simulink model "ofdm_pktdetector_mimo"  (Simulink 6.6)
settings: Solver=ode45  StartTime=0.0  StopTime=simTime  RelTol=1e-3
PreLoadFcn:
  | init
PostLoadFcn:
  | init
InitFcn:
  | init
StartFcn:
  | init
undefined symbols (not defined in the file or in its folder): gcbh, xlBlockLoadCallback, xlGetSimulinkPeriod
libraries: xbsIndex_r4 x201
(part 1 of 3)
settings Model: Creator=murphpo  LastModifiedBy=CMC
settings DebuggingCC: SignalResolutionControl=TryResolveAllWithWarning  MultiTaskDSMMsg=warning  MultiTaskCondExecSysMsg=none
settings RTWCC: IncludeERTFirstTime=on

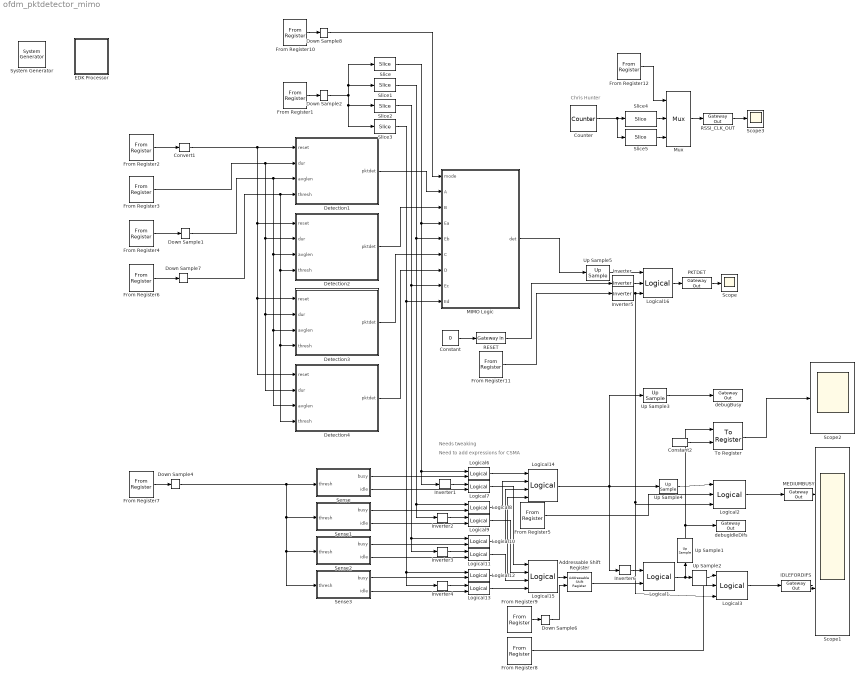
== system ofdm_pktdetector_mimo ==
  note: Chris Hunter
  note: Need to add expressions for CSMA
  note: Needs tweaking
  " System Generator" : xbsIndex_r4/ System Generator  Tag=genX  SystemSampleTime=-1  xilinxfamily=virtex2p  part=xc2vp70  speed=-6  package=ff1517  synthesis_tool=XST  clock_wrapper=Clock Enables  directory=./plb46_pktDet_v01  testbench=off  simulink_period=1/4  sysclk_period=10  dcm_input_clock_period=100  incr_netlist=off  trim_vbits=Everywhere in SubSystem  dbl_ovrd=According to Block Masks  core_generation=According to Block Masks  run_coregen=off  deprecated_control=off  eval_field=0  block_type=sysgen
      settings: block_version=8.2
  Addressable Shift Register : xbsIndex_r4/Addressable Shift Register  infer_latency=on  depth=2  initVector=[0]  en=off  dbl_ovrd=off  use_behavioral_HDL=off  use_rpm=off  block_type=addrsr
      settings: block_version=8.2
      settings: infoedit=|
      | Delay of  configurable length.  Any element  in the delay
      |     line   can    be   addressed   and   driven    onto   the   output
      |     port.<P><P>Hardware  notes: Implemented  using SRL16s.
      |     If Virtex-4, Virtex-II or Spartan-3 devices are used, multiple SRLC16s are cascaded together.
  Constant : Constant  Value=0
  Constant2 : xbsIndex_r4/Constant  arith_type=Boolean  const=1  n_bits=1  bin_pt=0  explicit_period=off  period=1  equ=P=C  opselect=C  inp2=PCIN>>17  opr=+  inp1=P  carry=CIN  dbl_ovrd=off  block_type=constant
      settings: block_version=8.2
  Convert1 : xbsIndex_r4/Convert  arith_type=Boolean  n_bits=16  bin_pt=14  quantization=Truncate  overflow=Wrap  latency=0  dbl_ovrd=off  pipeline=off  block_type=convert
      settings: block_version=VER_STRING_GOES_HERE
  Counter : xbsIndex_r4/Counter  cnt_type=Free Running  cnt_to=Inf  operation=Up  start_count=0  cnt_by_val=1  arith_type=Unsigned  n_bits=2  bin_pt=0  load_pin=off  rst=off  en=off  explicit_period=on  period=2/4  dbl_ovrd=off  use_behavioral_HDL=off  use_rpm=off  block_type=counter
      settings: block_version=VER_STRING_GOES_HERE
  Detection1 : Subsystem
  Detection2 : Subsystem
  Detection3 : Subsystem
  Detection4 : Subsystem
  Down Sample{1..2,4,6..8} (6 alike) : xbsIndex_r4/Down Sample  sample_ratio=4  sample_phase="Last Value of Frame  (most efficient)"  en=off  latency=1  dbl_ovrd=off  block_type=dsamp
      settings: block_version=VER_STRING_GOES_HERE
  EDK Processor : Subsystem  LoadFcn=xlBlockLoadCallback(gcbh);  mask(Xilinx EDK Processor Block){mode=EDK pcore generation, xmp=, MemVisToProc=<qt bgcolor="#FFFFFF"><div><img src="C:\Xilinx_101\DSP_Tools\common\bin\..\..\sysgen\data\images\registerplus.gif"> &lt;&lt;csma_avgThresh&gt;&gt;<br></div><div><img src="C:\Xilinx_101\DSP_Tools\common\bin\..\..\sysgen\data\images\registerplus.gif"> &lt;&lt;csma_difsPeriod&gt;&gt;<br></div><div><img src="C:\Xilinx_101\DSP_Tools\common\bin\..\..\sysgen\data\images\registerplus.gif"> &lt;&lt;csma_enableBusy&gt;&gt;<br></div><div><img src="C:\Xilinx_101\DSP_Tools\common\bin\..\..\sysgen\data\images\registerplus.gif"> &lt;&lt;csma_enableIdle&gt;&gt;<br></div><div><img src="C:\Xilinx_101\DSP_Tools\common\bin\..\..\sysgen\data\images\registerplus.gif"> &lt;&lt;pktDet_avgLen&gt;&gt;<br></div><div><img src="C:\Xilinx_101\DSP_Tools\common\bin\..\..\sysgen\data\images\registerplus.gif"> &lt;&lt;pktDet_avgThresh&gt;&gt;<br></div><div><img src="C:\Xilinx_101\DSP_Tools\common\bin\..\..\sysgen\data\images\registerplus.gif"> &lt;&lt;pktDet_clkRatioSel&gt;&gt;<br></div><div><img src="C:\Xilinx_101\DSP_Tools\common\bin\..\..\sysgen\data\images\registerplus.gif"> &lt;&lt;pktDet_detectionMask&gt;&gt;<br></div><div><img src="C:\Xilinx_101\DSP_Tools\common\bin\..\..\sysgen\data\images\registerplus.gif"> &lt;&lt;pktDet_detectionMode&gt;&gt;<br></div><div><img src="C:\Xilinx_101\DSP_Tools\common\bin\..\..\sysgen\data\images\registerplus.gif"> &lt;&lt;pktDet_idleDifs&gt;&gt;<br></div><div><img src="C:\Xilinx_101\DSP_Tools\common\bin\..\..\sysgen\data\images\registerplus.gif"> &lt;&lt;pktDet_masterReset&gt;&gt;<br></div><div><img src="C:\Xilinx_101\DSP_Tools\common\bin\..\..\sysgen\data\images\registerplus.gif"> &lt;&lt;pktDet_reset&gt;&gt;<br></div><div><img src="C:\Xilinx_101\DSP_Tools\common\bin\..\..\sysgen\data\images\registerplus.gif"> &lt;&lt;pktDet_resetDuration&gt;&gt;<br></div></qt>, AvailableMemories=<empty>, portInterfaceTable={'exposed'=>[],'portdir'=>[],'portname'=>[],'shortname'=>[]}, bus_type_sgadvanced=, bus_type=PLB, baseaddr=0x80000000, baseaddr_lock_sgadvanced=, baseaddr_lock=off, dual_clock_sgadvanced=, dual_clock=off, ucf_file=, inheritDeviceType_sgadvanced=, inheritDeviceType=off, clock_name=plb, internalPortList={}, resetPolarity=0, memxtable={'mlist'=>['ofdm_pktdetector_mimo/From Register7','ofdm_pktdetector_mimo/From Register9','ofdm_pktdetector_mimo/From Register5','ofdm_pktdetector_mimo/From Register8','ofdm_pktdetector_mimo/From Register4','ofdm_pktdetector_mimo/From Register6','ofdm_pktdetector_mimo/From Register12','ofdm_pktdetector_mimo/From Register1','ofdm_pktdetector_mimo/From Register10','ofdm_pktdetector_mimo/To Register','ofdm_pktdetector_mimo/From Register2','ofdm_pktdetector_mimo/From Register11','ofdm_pktdetector_mimo/From Register3'],'mlname'=>['\'csma_avgThresh\'','\'csma_difsPeriod\'','\'csma_enableBusy\'','\'csma_enableIdle\'','\'pktDet_avgLen\'','\'pktDet_avgThresh\'','\'pktDet_clkRatioSel\'','\'pktDet_detectionMask\'','\'pktDet_detectionMode\'','\'pktDet_idleDifs\'','\'pktDet_masterReset\'','\'pktDet_reset\'','\'pktDet_resetDuration\''],'mlstate'=>[0.00000000000000000,0.00000000000000000,0.00000000000000000,0.00000000000000000,0.00000000000000000,0.00000000000000000,0.00000000000000000,0.00000000000000000,0.00000000000000000,0.00000000000000000,0.00000000000000000,0.00000000000000000,0.00000000000000000]}, procinfo={'xmliface'=>'Xilinx//microblaze//iface.xml'}, fslifaceports=[0,0], memmapdirty=off, blockname=, xpsintstyle=default, proc=, has_advanced_control=0, sggui_pos=20,20,383,441, block_type=edkprocessor, block_version=2.4, sg_icon_stat=62,64,-1,-1,white,blue,0,07734,right, sg_mask_display=|, sg_list_contents={'table'=>{'AvailableMemories'=>'popup(<empty>)','userSelections'=>{'AvailableMemories'=>'<empty>'}}}, sg_blockgui_xml=}
      mask sg_mask_display=|
      | fprintf('','COMMENT: begin icon graphics');
      | patch([0 62 62 0 ],[0 0 64 64 ],[0.77 0.82 0.91]);
      | patch([14 4 19 4 14 30 34 38 56 42 29 19 33 19 29 42 56 38 34 30 14 ],[8 18 33 48 58 58 54 58 58 44 57 47 33 19 9 22 8 8 12 8 8 ],[0.98 0.96 0.92]);
      | plot([0 62 62 0 0 ],[0 0 64 64 0 ]);
      | fprintf('','COMMENT: end icon graphics');
      | fprintf('','COMMENT: begin icon text');
      | fprintf('','COMMENT: end icon text');
      mask prompts: mode "Configure Processor for"; xmp "EDK Project"; MemVisToProc ""; AvailableMemories "Available Memories"; portInterfaceTable ""; bus_type_sgadvanced ""; bus_type "Bus Type"; baseaddr "Base Address"; baseaddr_lock_sgadvanced ""; baseaddr_lock "Lock"; dual_clock_sgadvanced ""; dual_clock "Dual Clocks"; ucf_file "Constraint file"; inheritDeviceType_sgadvanced ""; inheritDeviceType "Inherit Device Type"; clock_name ""; internalPortList ""; resetPolarity ""; memxtable ""; procinfo ""; fslifaceports ""; memmapdirty ""; blockname ""; xpsintstyle ""; proc ""; has_advanced_control ""; sggui_pos ""; block_type ""; block_version ""; sg_icon_stat ""; sg_mask_display ""; sg_list_contents ""; sg_blockgui_xml ""
      mask help: Xilinx EDK Processor
      mask init:
      | try
      |   tmp_gcb = gcb;
      |   tmp_gcbh = gcbh;
      |   if (strcmp('SysGenIndex',get_param(bdroot(tmp_gcbh),'tag')) && ~isempty(regexp(bdroot(tmp_gcb), '^xbs', 'once')))
      |     return;
      |   end;
      |   xlMungeMaskParams;
      |   serialized_declarations = '{}';
      |   xledkprocessor_init();
      |   ptable_ = xlblockprep(get_param(tmp_gcb, 'MaskWSVariables'));
      | catch
      |   global dbgsysgen;
      |   if(~isempty(dbgsysgen) && dbgsysgen)
      |     e = regexprep(lasterr, '\n', '\nError: ');
      |     disp(['Error: While running MaskInit code on block ' tmp_gcb ': ' e]);
      |     error(e);
      |   end
      | end
      settings: CopyFcn=xlProcBlockCopyCallback(gcbh);xlBlockMoveCallback(gcbh);  DeleteFcn=xlDestroyGui(gcbh);  ModelCloseFcn=xlDestroyGui(gcbh);  PreSaveFcn=xlBlockPreSaveCallback(gcbh);  PostSaveFcn=xlBlockPostSaveCallback(gcbh);  DestroyFcn=xlDestroyGui(gcbh);  OpenFcn=bh=gcbh;xlProcBlockCallbacks('populatesharedmemorylistbox',bh);xlOpenGui(bh, 'edkprocessor_gui.xml', @xlProcBlockEnablement, @xlProcBlockAction)  CloseFcn=xlDestroyGui(gcbh);  MoveFcn=xlBlockMoveCallback(gcbh);
      mask Help: eval('');xlDoc('-book','sysgen','-topic','EDK_Processor');
      mask StyleString: popup(EDK pcore generation|HDL netlisting),edit,edit,popup(<empty>),edit,edit,popup(PLB|FSL),edit,edit,checkbox,edit,checkbox,edit,edit,checkbox,edit,edit,edit,edit,edit,edit,edit,edit,edit,edit,edit,edit,edit,edit,edit,edit,edit,edit
      mask Display:
      | fprintf('','COMMENT: begin icon graphics');
      | patch([0 62 62 0 ],[0 0 64 64 ],[0.77 0.82 0.91]);
      | patch([14 4 19 4 14 30 34 38 56 42 29 19 33 19 29 42 56 38 34 30 14 ],[8 18 33 48 58 58 54 58 58 44 57 47 33 19 9 22 8 8 12 8 8 ],[0.98 0.96 0.92]);
      | plot([0 62 62 0 0 ],[0 0 64 64 0 ]);
      | fprintf('','COMMENT: end icon graphics');
      | fprintf('','COMMENT: begin icon text');
      | disp('MicroBlaze');
      | 
      | fprintf('','COMMENT: end icon text');
  From Register1 : xbsIndex_r4/From Register  shared_memory_name='pktDet_detectionMask'  init=3  period=1/4  ownership=Locally owned and initialized  arith_type=Unsigned  n_bits=4  bin_pt=0  dbl_ovrd=off  block_type=fromreg
      settings: AttributesFormatString=From Register\n<< %<shared_memory_name> >>  infoedit="Register block that reads data to a shared memory register.  Delay of one sample period."  block_version=8.2
  From Register10 : xbsIndex_r4/From Register  shared_memory_name='pktDet_detectionMode'  init=1  period=1/4  ownership=Locally owned and initialized  arith_type=Unsigned  n_bits=1  bin_pt=0  dbl_ovrd=off  block_type=fromreg
      settings: AttributesFormatString=From Register\n<< %<shared_memory_name> >>  infoedit="Register block that reads data to a shared memory register.  Delay of one sample period."  block_version=8.2
  From Register11 : xbsIndex_r4/From Register  shared_memory_name='pktDet_reset'  init=0  period=1/4  ownership=Locally owned and initialized  arith_type=Unsigned  n_bits=1  bin_pt=0  dbl_ovrd=off  block_type=fromreg
      settings: AttributesFormatString=From Register\n<< %<shared_memory_name> >>  infoedit="Register block that reads data to a shared memory register.  Delay of one sample period."  block_version=8.2
  From Register12 : xbsIndex_r4/From Register  shared_memory_name='pktDet_clkRatioSel'  init=0  period=1/4  ownership=Locally owned and initialized  arith_type=Unsigned  n_bits=1  bin_pt=0  dbl_ovrd=off  block_type=fromreg
      settings: AttributesFormatString=From Register\n<< %<shared_memory_name> >>  infoedit="Register block that reads data to a shared memory register.  Delay of one sample period."  block_version=8.2
  From Register2 : xbsIndex_r4/From Register  shared_memory_name='pktDet_masterReset'  init=0  period=1/4  ownership=Locally owned and initialized  arith_type=Unsigned  n_bits=1  bin_pt=0  dbl_ovrd=off  block_type=fromreg
      settings: AttributesFormatString=From Register\n<< %<shared_memory_name> >>  infoedit="Register block that reads data to a shared memory register.  Delay of one sample period."  block_version=8.2
  From Register3 : xbsIndex_r4/From Register  shared_memory_name='pktDet_resetDuration'  init=resetDuration  period=1/4  ownership=Locally owned and initialized  arith_type=Unsigned  n_bits=16  bin_pt=0  dbl_ovrd=off  block_type=fromreg
      settings: AttributesFormatString=From Register\n<< %<shared_memory_name> >>  infoedit="Register block that reads data to a shared memory register.  Delay of one sample period."  block_version=8.2
  From Register4 : xbsIndex_r4/From Register  shared_memory_name='pktDet_avgLen'  init=2^5  period=1/4  ownership=Locally owned and initialized  arith_type=Unsigned  n_bits=5  bin_pt=0  dbl_ovrd=off  block_type=fromreg
      settings: AttributesFormatString=From Register\n<< %<shared_memory_name> >>  infoedit="Register block that reads data to a shared memory register.  Delay of one sample period."  block_version=8.2
  From Register5 : xbsIndex_r4/From Register  shared_memory_name='csma_enableBusy'  init=1  period=1/4  ownership=Locally owned and initialized  arith_type=Unsigned  n_bits=1  bin_pt=0  dbl_ovrd=off  block_type=fromreg
      settings: AttributesFormatString=From Register\n<< %<shared_memory_name> >>  infoedit="Register block that reads data to a shared memory register.  Delay of one sample period."  block_version=8.2
  From Register6 : xbsIndex_r4/From Register  shared_memory_name='pktDet_avgThresh'  init=avgMode_avgThresh  period=1/4  ownership=Locally owned and initialized  arith_type=Unsigned  n_bits=16  bin_pt=0  dbl_ovrd=off  block_type=fromreg
      settings: AttributesFormatString=From Register\n<< %<shared_memory_name> >>  infoedit="Register block that reads data to a shared memory register.  Delay of one sample period."  block_version=8.2
  From Register7 : xbsIndex_r4/From Register  shared_memory_name='csma_avgThresh'  init=avgMode_avgThresh  period=1/4  ownership=Locally owned and initialized  arith_type=Unsigned  n_bits=16  bin_pt=0  dbl_ovrd=off  block_type=fromreg
      settings: AttributesFormatString=From Register\n<< %<shared_memory_name> >>  infoedit="Register block that reads data to a shared memory register.  Delay of one sample period."  block_version=8.2
  From Register8 : xbsIndex_r4/From Register  shared_memory_name='csma_enableIdle'  init=1  period=1/4  ownership=Locally owned and initialized  arith_type=Unsigned  n_bits=1  bin_pt=0  dbl_ovrd=off  block_type=fromreg
      settings: AttributesFormatString=From Register\n<< %<shared_memory_name> >>  infoedit="Register block that reads data to a shared memory register.  Delay of one sample period."  block_version=8.2
  From Register9 : xbsIndex_r4/From Register  shared_memory_name='csma_difsPeriod'  init=625  period=1/4  ownership=Locally owned and initialized  arith_type=Unsigned  n_bits=10  bin_pt=0  dbl_ovrd=off  block_type=fromreg
      settings: AttributesFormatString=From Register\n<< %<shared_memory_name> >>  infoedit="Register block that reads data to a shared memory register.  Delay of one sample period."  block_version=8.2
  IDLEFORDIFS : xbsIndex_r4/Gateway Out  hdl_port=on  timing_constraint=None  locs_specified=off  LOCs={}  block_type=gatewayout
      settings: infoedit="Gateway out block.  Converts Xilinx fixed point inputs into ouputs of type Simulink integer, double, or fixed point.<P><P>Hardware notes:  In hardware these blocks become top level output ports or are discarded, depending on how they are configured."  block_version=VER_STRING_GOES_HERE
  Inverter{,1..6} (7 alike) : xbsIndex_r4/Inverter  en=off  latency=0  dbl_ovrd=off  block_type=inv
      settings: block_version=8.2
  Logical{1,6,8,10,12} (5 alike) : xbsIndex_r4/Logical  logical_function=AND  inputs=2  en=off  latency=0  precision=Full  arith_type=Unsigned  n_bits=16  bin_pt=0  align_bp=on  dbl_ovrd=off  block_type=logical
      settings: block_version=8.2
  Logical{7,9,11,13} (4 alike) : xbsIndex_r4/Logical  logical_function=OR  inputs=2  en=off  latency=0  precision=Full  arith_type=Unsigned  n_bits=16  bin_pt=0  align_bp=on  dbl_ovrd=off  block_type=logical
      settings: block_version=8.2
  Logical14 : xbsIndex_r4/Logical  logical_function=OR  inputs=4  en=off  latency=0  precision=Full  arith_type=Unsigned  n_bits=16  bin_pt=0  align_bp=on  dbl_ovrd=off  block_type=logical
      settings: block_version=8.2
  Logical15 : xbsIndex_r4/Logical  logical_function=AND  inputs=4  en=off  latency=0  precision=Full  arith_type=Unsigned  n_bits=16  bin_pt=0  align_bp=on  dbl_ovrd=off  block_type=logical
      settings: block_version=8.2
  Logical16 : xbsIndex_r4/Logical  logical_function=AND  inputs=3  en=off  latency=0  precision=Full  arith_type=Unsigned  n_bits=16  bin_pt=0  align_bp=on  dbl_ovrd=off  block_type=logical
      settings: block_version=8.2
  Logical2 : xbsIndex_r4/Logical  logical_function=AND  inputs=3  en=off  latency=0  precision=Full  arith_type=Unsigned  n_bits=16  bin_pt=0  align_bp=on  dbl_ovrd=off  block_type=logical
      settings: block_version=8.2
  Logical3 : xbsIndex_r4/Logical  logical_function=AND  inputs=3  en=off  latency=0  precision=Full  arith_type=Unsigned  n_bits=16  bin_pt=0  align_bp=on  dbl_ovrd=off  block_type=logical
      settings: block_version=8.2
  MEDIUMBUSY : xbsIndex_r4/Gateway Out  hdl_port=on  timing_constraint=None  locs_specified=off  LOCs={}  block_type=gatewayout
      settings: infoedit="Gateway out block.  Converts Xilinx fixed point inputs into ouputs of type Simulink integer, double, or fixed point.<P><P>Hardware notes:  In hardware these blocks become top level output ports or are discarded, depending on how they are configured."  block_version=VER_STRING_GOES_HERE
  MIMO Logic : Subsystem
  Mux : xbsIndex_r4/Mux  inputs=2  en=off  latency=0  precision=Full  arith_type=Unsigned  n_bits=16  bin_pt=14  quantization=Truncate  overflow=Wrap  dbl_ovrd=off  block_type=mux
      settings: block_version=8.2.02
  PKTDET : xbsIndex_r4/Gateway Out  hdl_port=on  timing_constraint=None  locs_specified=off  LOCs={}  block_type=gatewayout
      settings: infoedit="Gateway out block.  Converts Xilinx fixed point inputs into ouputs of type Simulink integer, double, or fixed point.<P><P>Hardware notes:  In hardware these blocks become top level output ports or are discarded, depending on how they are configured."  block_version=VER_STRING_GOES_HERE
  RESET : xbsIndex_r4/Gateway In  arith_type=Unsigned  n_bits=1  bin_pt=0  quantization="Round  (unbiased: +/- Inf)"  overflow=Saturate  period=1/4  dbl_ovrd=off  timing_constraint=None  locs_specified=off  LOCs={}  block_type=gatewayin
      settings: infoedit="Gateway in block.  Converts inputs of type Simulink integer, double and fixed point to  Xilinx fixed point type.<P><P>Hardware notes:  In hardware these blocks become top level input ports."  block_version=VER_STRING_GOES_HERE
  RSSI_CLK_OUT : xbsIndex_r4/Gateway Out  hdl_port=on  timing_constraint=None  locs_specified=off  LOCs={}  block_type=gatewayout
      settings: infoedit="Gateway out block.  Converts Xilinx fixed point inputs into ouputs of type Simulink integer, double, or fixed point.<P><P>Hardware notes:  In hardware these blocks become top level output ports or are discarded, depending on how they are configured."  block_version=VER_STRING_GOES_HERE
  Scope : Scope
  Scope1 : Scope  NumInputPorts=2
      settings: YMin=-5~-5  YMax=5~5  SaveName=ScopeData2
  Scope2 : Scope
      settings: SaveName=ScopeData4
  Scope3 : Scope
      settings: SaveName=ScopeData3
  Sense : Subsystem
  Sense1 : Subsystem
  Sense2 : Subsystem
  Sense3 : Subsystem
  Slice : xbsIndex_r4/Slice  nbits=1  boolean_output=off  mode=Lower Bit Location + Width  bit1=0  base1=MSB of Input  bit0=0  base0=LSB of Input  dbl_ovrd=off  block_type=slice
      settings: infoedit="Extracts a given range of bits from each input sample and presents it at the output.  The output type is ordinarily unsigned with binary point at zero, but can be Boolean when the slice is one bit wide.<P><P>Hardware notes: In hardware this block costs nothing."  block_version=8.2
  Slice1 : xbsIndex_r4/Slice  nbits=1  boolean_output=off  mode=Lower Bit Location + Width  bit1=0  base1=MSB of Input  bit0=1  base0=LSB of Input  dbl_ovrd=off  block_type=slice
      settings: infoedit="Extracts a given range of bits from each input sample and presents it at the output.  The output type is ordinarily unsigned with binary point at zero, but can be Boolean when the slice is one bit wide.<P><P>Hardware notes: In hardware this block costs nothing."  block_version=8.2
  Slice2 : xbsIndex_r4/Slice  nbits=1  boolean_output=off  mode=Lower Bit Location + Width  bit1=0  base1=MSB of Input  bit0=2  base0=LSB of Input  dbl_ovrd=off  block_type=slice
      settings: infoedit="Extracts a given range of bits from each input sample and presents it at the output.  The output type is ordinarily unsigned with binary point at zero, but can be Boolean when the slice is one bit wide.<P><P>Hardware notes: In hardware this block costs nothing."  block_version=8.2
  Slice3 : xbsIndex_r4/Slice  nbits=1  boolean_output=off  mode=Lower Bit Location + Width  bit1=0  base1=MSB of Input  bit0=3  base0=LSB of Input  dbl_ovrd=off  block_type=slice
      settings: infoedit="Extracts a given range of bits from each input sample and presents it at the output.  The output type is ordinarily unsigned with binary point at zero, but can be Boolean when the slice is one bit wide.<P><P>Hardware notes: In hardware this block costs nothing."  block_version=8.2
  Slice4 : xbsIndex_r4/Slice  nbits=1  boolean_output=off  mode=Lower Bit Location + Width  bit1=0  base1=MSB of Input  bit0=0  base0=LSB of Input  dbl_ovrd=off  block_type=slice
      settings: infoedit="Extracts a given range of bits from each input sample and presents it at the output.  The output type is ordinarily unsigned with binary point at zero, but can be Boolean when the slice is one bit wide.<P><P>Hardware notes: In hardware this block costs nothing."  block_version=8.2.02
  Slice5 : xbsIndex_r4/Slice  nbits=1  boolean_output=off  mode=Upper Bit Location + Width  bit1=0  base1=MSB of Input  bit0=0  base0=LSB of Input  dbl_ovrd=off  block_type=slice
      settings: infoedit="Extracts a given range of bits from each input sample and presents it at the output.  The output type is ordinarily unsigned with binary point at zero, but can be Boolean when the slice is one bit wide.<P><P>Hardware notes: In hardware this block costs nothing."  block_version=8.2.02
  To Register : xbsIndex_r4/To Register  shared_memory_name='pktDet_idleDifs'  init=0  ownership=Locally owned and initialized  explicit_data_type=on  arith_type=Unsigned  n_bits=1  bin_pt=0  dbl_ovrd=off  block_type=toreg
      settings: AttributesFormatString=To Register\n<< %<shared_memory_name> >>  infoedit="Register block that writes data to a shared memory register.  Delay of one sample period."  block_version=8.2
  Up Sample1 : xbsIndex_r4/Up Sample  Orientation=up  sample_ratio=4  copy_samples=on  dbl_ovrd=off  block_type=usamp
      settings: infoedit="Up samples input data.  Inserted values  can be zeros or copies of the most recent input sample.<P><P>Hardware notes: No hardware is needed if inserted values are copies of the input sample; otherwise, a mux and single bit flip-flop are used."  block_version=8.2
  Up Sample{2..5} (4 alike) : xbsIndex_r4/Up Sample  sample_ratio=4  copy_samples=on  dbl_ovrd=off  block_type=usamp
      settings: infoedit="Up samples input data.  Inserted values  can be zeros or copies of the most recent input sample.<P><P>Hardware notes: No hardware is needed if inserted values are copies of the input sample; otherwise, a mux and single bit flip-flop are used."  block_version=8.2
  debugBusy : xbsIndex_r4/Gateway Out  hdl_port=on  timing_constraint=None  locs_specified=off  LOCs={}  block_type=gatewayout
      settings: infoedit="Gateway out block.  Converts Xilinx fixed point inputs into ouputs of type Simulink integer, double, or fixed point.<P><P>Hardware notes:  In hardware these blocks become top level output ports or are discarded, depending on how they are configured."  block_version=VER_STRING_GOES_HERE
  debugIdleDifs : xbsIndex_r4/Gateway Out  hdl_port=on  timing_constraint=None  locs_specified=off  LOCs={}  block_type=gatewayout
      settings: infoedit="Gateway out block.  Converts Xilinx fixed point inputs into ouputs of type Simulink integer, double, or fixed point.<P><P>Hardware notes:  In hardware these blocks become top level output ports or are discarded, depending on how they are configured."  block_version=VER_STRING_GOES_HERE
  wires:
  From Register4/1 -> Down Sample1/1
  RSSI_CLK_OUT/1 -> Scope3/1
  From Register2/1 -> Convert1/1
  From Register6/1 -> Down Sample7/1
  Convert1/1 -> Detection1/1(reset), Detection3/1(reset), Detection4/1(reset), Detection2/1(reset)
  From Register3/1 -> Detection1/2(dur), Detection3/2(dur), Detection4/2(dur), Detection2/2(dur)
  Down Sample1/1 -> Detection1/3(avglen), Detection3/3(avglen), Detection4/3(avglen), Detection2/3(avglen)
  Down Sample7/1 -> Detection1/4(thresh), Detection3/4(thresh), Detection4/4(thresh), Detection2/4(thresh)
  From Register1/1 -> Down Sample2/1
  Down Sample2/1 -> Slice/1, Slice1/1, Slice2/1, Slice3/1
  MIMO Logic/1(det) -> Up Sample5/1
  Slice/1 -> Logical6/1, Inverter1/1, MIMO Logic/4(Ea)
  Slice1/1 -> Logical8/1, Inverter2/1, MIMO Logic/5(Eb)
  Slice2/1 -> Logical10/1, Inverter3/1, MIMO Logic/8(Ec)
  Slice3/1 -> Logical12/1, Inverter4/1, MIMO Logic/9(Ed)
  PKTDET/1 -> Scope/1
  RESET/1 -> Inverter/1
  Constant/1 -> RESET/1
  Up Sample5/1 -> Logical16/1
  Logical16/1 -> PKTDET/1
  From Register7/1 -> Down Sample4/1
  Down Sample4/1 -> Sense/1(thresh), Sense2/1(thresh), Sense3/1(thresh), Sense1/1(thresh)
  Sense/1(busy) -> Logical6/2
  Sense/2(idle) -> Logical7/2
  Sense1/1(busy) -> Logical8/2
  Sense1/2(idle) -> Logical9/2
  Sense2/1(busy) -> Logical10/2
  Sense2/2(idle) -> Logical11/2
  Sense3/1(busy) -> Logical12/2
  Sense3/2(idle) -> Logical13/2
  Logical6/1 -> Logical14/1
  Logical8/1 -> Logical14/2
  Logical10/1 -> Logical14/3
  Logical12/1 -> Logical14/4
  Logical13/1 -> Logical15/4
  Logical11/1 -> Logical15/3
  Logical9/1 -> Logical15/2
  Logical7/1 -> Logical15/1
  Logical14/1 -> Inverter6/1, Up Sample4/1, Up Sample3/1
  From Register5/1 -> Logical2/2
  From Register8/1 -> Logical3/2
  Logical15/1 -> Addressable Shift Register/1
  From Register9/1 -> Down Sample6/1
  Down Sample6/1 -> Addressable Shift Register/2
  Logical2/1 -> MEDIUMBUSY/1
  Inverter/1 -> Logical16/2
  MEDIUMBUSY/1 -> Scope1/1
  IDLEFORDIFS/1 -> Scope1/2
  Inverter4/1 -> Logical13/1
  Inverter3/1 -> Logical11/1
  Inverter2/1 -> Logical9/1
  Inverter1/1 -> Logical7/1
  Detection1/1(pktdet) -> MIMO Logic/2(A)
  Detection3/1(pktdet) -> MIMO Logic/6(C)
  From Register10/1 -> Down Sample8/1
  Detection2/1(pktdet) -> MIMO Logic/3(B)
  Detection4/1(pktdet) -> MIMO Logic/7(D)
  From Register11/1 -> Inverter5/1
  Inverter5/1 -> Logical16/3, Logical2/3, Logical3/3
  Down Sample8/1 -> MIMO Logic/1(mode)
  Logical1/1 -> Up Sample2/1, Up Sample1/1
  Addressable Shift Register/1 -> Logical1/2
  Inverter6/1 -> Logical1/1
  Constant2/1 -> To Register/2
  Up Sample4/1 -> Logical2/1
  Up Sample2/1 -> Logical3/1
  Logical3/1 -> IDLEFORDIFS/1
  To Register/1 -> Scope2/1
  Up Sample3/1 -> debugBusy/1
  Up Sample1/1 -> debugIdleDifs/1, To Register/1
  Mux/1 -> RSSI_CLK_OUT/1
  Counter/1 -> Slice4/1, Slice5/1
  Slice4/1 -> Mux/2
  Slice5/1 -> Mux/3
  From Register12/1 -> Mux/1

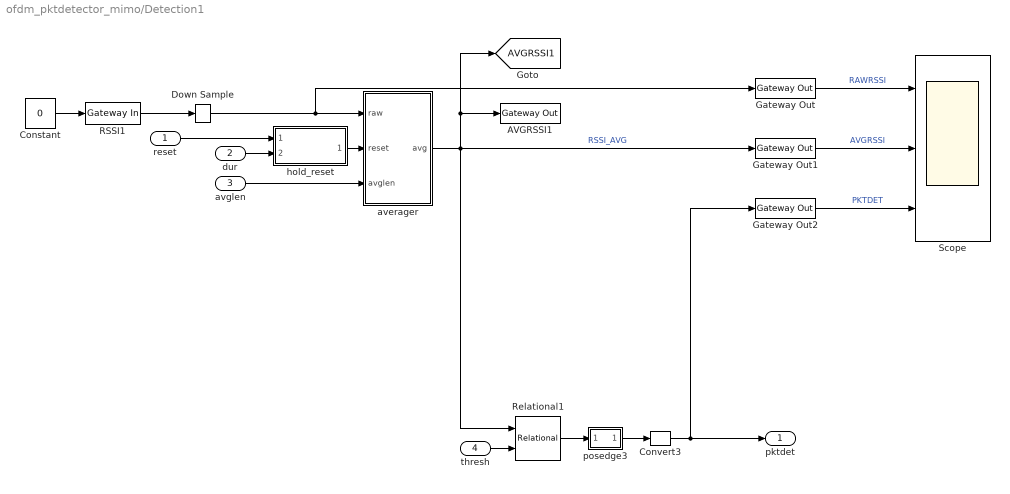
== system ofdm_pktdetector_mimo/Detection1 ==
  reset : Inport
  dur : Inport  Port=2
  avglen : Inport  Port=3
  thresh : Inport  Port=4
  AVGRSSI1 : xbsIndex_r4/Gateway Out  hdl_port=on  timing_constraint=None  locs_specified=off  LOCs={}  block_type=gatewayout
      settings: infoedit="Gateway out block.  Converts Xilinx fixed point inputs into ouputs of type Simulink integer, double, or fixed point.<P><P>Hardware notes:  In hardware these blocks become top level output ports or are discarded, depending on how they are configured."  block_version=8.2
  Constant : Constant  Value=0
  Convert3 : xbsIndex_r4/Convert  arith_type=Unsigned  n_bits=1  bin_pt=0  quantization=Truncate  overflow=Wrap  latency=0  dbl_ovrd=off  pipeline=off  block_type=convert
      settings: block_version=VER_STRING_GOES_HERE
  Down Sample : xbsIndex_r4/Down Sample  sample_ratio=4  sample_phase="Last Value of Frame  (most efficient)"  en=off  latency=1  dbl_ovrd=off  block_type=dsamp
      settings: block_version=VER_STRING_GOES_HERE
  Gateway Out : xbsIndex_r4/Gateway Out  hdl_port=off  timing_constraint=None  locs_specified=off  LOCs={}  block_type=gatewayout
      settings: infoedit="Gateway out block.  Converts Xilinx fixed point inputs into ouputs of type Simulink integer, double, or fixed point.<P><P>Hardware notes:  In hardware these blocks become top level output ports or are discarded, depending on how they are configured."  block_version=8.2
  Gateway Out1 : xbsIndex_r4/Gateway Out  hdl_port=off  timing_constraint=None  locs_specified=off  LOCs={}  block_type=gatewayout
      settings: infoedit="Gateway out block.  Converts Xilinx fixed point inputs into ouputs of type Simulink integer, double, or fixed point.<P><P>Hardware notes:  In hardware these blocks become top level output ports or are discarded, depending on how they are configured."  block_version=8.2
  Gateway Out2 : xbsIndex_r4/Gateway Out  hdl_port=off  timing_constraint=None  locs_specified=off  LOCs={}  block_type=gatewayout
      settings: infoedit="Gateway out block.  Converts Xilinx fixed point inputs into ouputs of type Simulink integer, double, or fixed point.<P><P>Hardware notes:  In hardware these blocks become top level output ports or are discarded, depending on how they are configured."  block_version=8.2
  RSSI1 : xbsIndex_r4/Gateway In  arith_type=Unsigned  n_bits=10  bin_pt=0  quantization="Round  (unbiased: +/- Inf)"  overflow=Saturate  period=1/4  dbl_ovrd=off  timing_constraint=None  locs_specified=off  LOCs={}  block_type=gatewayin
      settings: infoedit="Gateway in block.  Converts inputs of type Simulink integer, double and fixed point to  Xilinx fixed point type.<P><P>Hardware notes:  In hardware these blocks become top level input ports."  block_version=VER_STRING_GOES_HERE
  Relational1 : xbsIndex_r4/Relational  mode=a>b  en=off  latency=0  dbl_ovrd=off  block_type=relational
      settings: block_version=VER_STRING_GOES_HERE
  Scope : Scope  NumInputPorts=3
      settings: YMin=-1~-1~-1  YMax=1~1~1
  averager : Subsystem
  hold_reset : Subsystem
  posedge3 : Subsystem
  pktdet : Outport
  tag scope: AVGRSSI1=global
  wires:
  averager/1(avg) -> Relational1/1, Gateway Out1/1, AVGRSSI1/1, [AVGRSSI1]  "RSSI_AVG"
  hold_reset/1(reset_out) -> averager/2(reset)
  Relational1/1 -> posedge3/1(In)
  posedge3/1(Out) -> Convert3/1
  dur/1 -> hold_reset/2(duration)
  reset/1 -> hold_reset/1(reset_in)
  avglen/1 -> averager/3(avglen)
  Convert3/1 -> pktdet/1, Gateway Out2/1
  thresh/1 -> Relational1/2
  RSSI1/1 -> Down Sample/1
  Down Sample/1 -> averager/1(raw), Gateway Out/1
  Constant/1 -> RSSI1/1
  Gateway Out/1 -> Scope/1  "RAWRSSI"
  Gateway Out1/1 -> Scope/2  "AVGRSSI"
  Gateway Out2/1 -> Scope/3  "PKTDET"

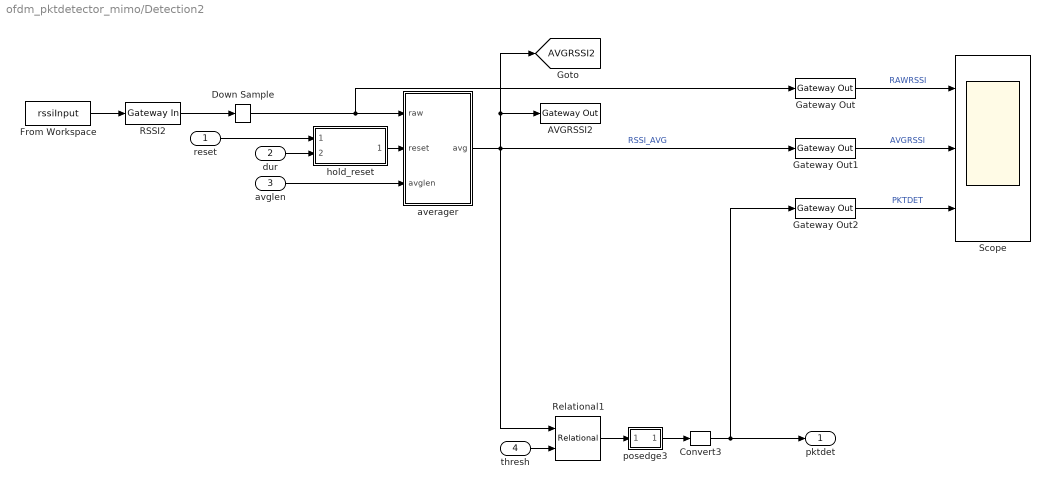
== system ofdm_pktdetector_mimo/Detection2 ==
  reset : Inport
  dur : Inport  Port=2
  avglen : Inport  Port=3
  thresh : Inport  Port=4
  AVGRSSI2 : xbsIndex_r4/Gateway Out  hdl_port=on  timing_constraint=None  locs_specified=off  LOCs={}  block_type=gatewayout
      settings: infoedit="Gateway out block.  Converts Xilinx fixed point inputs into ouputs of type Simulink integer, double, or fixed point.<P><P>Hardware notes:  In hardware these blocks become top level output ports or are discarded, depending on how they are configured."  block_version=8.2
  Convert3 : xbsIndex_r4/Convert  arith_type=Unsigned  n_bits=1  bin_pt=0  quantization=Truncate  overflow=Wrap  latency=0  dbl_ovrd=off  pipeline=off  block_type=convert
      settings: block_version=VER_STRING_GOES_HERE
  Down Sample : xbsIndex_r4/Down Sample  sample_ratio=4  sample_phase="Last Value of Frame  (most efficient)"  en=off  latency=1  dbl_ovrd=off  block_type=dsamp
      settings: block_version=VER_STRING_GOES_HERE
  From Workspace : FromWorkspace  VariableName=rssiInput  SampleTime=1/4  Interpolate=off  OutputAfterFinalValue=Setting to zero
  Gateway Out : xbsIndex_r4/Gateway Out  hdl_port=off  timing_constraint=None  locs_specified=off  LOCs={}  block_type=gatewayout
      settings: infoedit="Gateway out block.  Converts Xilinx fixed point inputs into ouputs of type Simulink integer, double, or fixed point.<P><P>Hardware notes:  In hardware these blocks become top level output ports or are discarded, depending on how they are configured."  block_version=8.2
  Gateway Out1 : xbsIndex_r4/Gateway Out  hdl_port=off  timing_constraint=None  locs_specified=off  LOCs={}  block_type=gatewayout
      settings: infoedit="Gateway out block.  Converts Xilinx fixed point inputs into ouputs of type Simulink integer, double, or fixed point.<P><P>Hardware notes:  In hardware these blocks become top level output ports or are discarded, depending on how they are configured."  block_version=8.2
  Gateway Out2 : xbsIndex_r4/Gateway Out  hdl_port=off  timing_constraint=None  locs_specified=off  LOCs={}  block_type=gatewayout
      settings: infoedit="Gateway out block.  Converts Xilinx fixed point inputs into ouputs of type Simulink integer, double, or fixed point.<P><P>Hardware notes:  In hardware these blocks become top level output ports or are discarded, depending on how they are configured."  block_version=8.2
  RSSI2 : xbsIndex_r4/Gateway In  arith_type=Unsigned  n_bits=10  bin_pt=0  quantization="Round  (unbiased: +/- Inf)"  overflow=Saturate  period=1/4  dbl_ovrd=off  timing_constraint=None  locs_specified=off  LOCs={}  block_type=gatewayin
      settings: infoedit="Gateway in block.  Converts inputs of type Simulink integer, double and fixed point to  Xilinx fixed point type.<P><P>Hardware notes:  In hardware these blocks become top level input ports."  block_version=VER_STRING_GOES_HERE
  Relational1 : xbsIndex_r4/Relational  mode=a>b  en=off  latency=0  dbl_ovrd=off  block_type=relational
      settings: block_version=VER_STRING_GOES_HERE
  Scope : Scope  NumInputPorts=3
      settings: YMin=-1~-1~-1  YMax=1~1~1
  averager : Subsystem
  hold_reset : Subsystem
  posedge3 : Subsystem
  pktdet : Outport
  tag scope: AVGRSSI2=global
  wires:
  Gateway Out2/1 -> Scope/3  "PKTDET"
  Gateway Out1/1 -> Scope/2  "AVGRSSI"
  Gateway Out/1 -> Scope/1  "RAWRSSI"
  From Workspace/1 -> RSSI2/1
  Down Sample/1 -> Gateway Out/1, averager/1(raw)
  RSSI2/1 -> Down Sample/1
  thresh/1 -> Relational1/2
  Convert3/1 -> Gateway Out2/1, pktdet/1
  avglen/1 -> averager/3(avglen)
  reset/1 -> hold_reset/1(reset_in)
  dur/1 -> hold_reset/2(duration)
  posedge3/1(Out) -> Convert3/1
  Relational1/1 -> posedge3/1(In)
  hold_reset/1(reset_out) -> averager/2(reset)
  averager/1(avg) -> [AVGRSSI2], AVGRSSI2/1, Gateway Out1/1, Relational1/1  "RSSI_AVG"

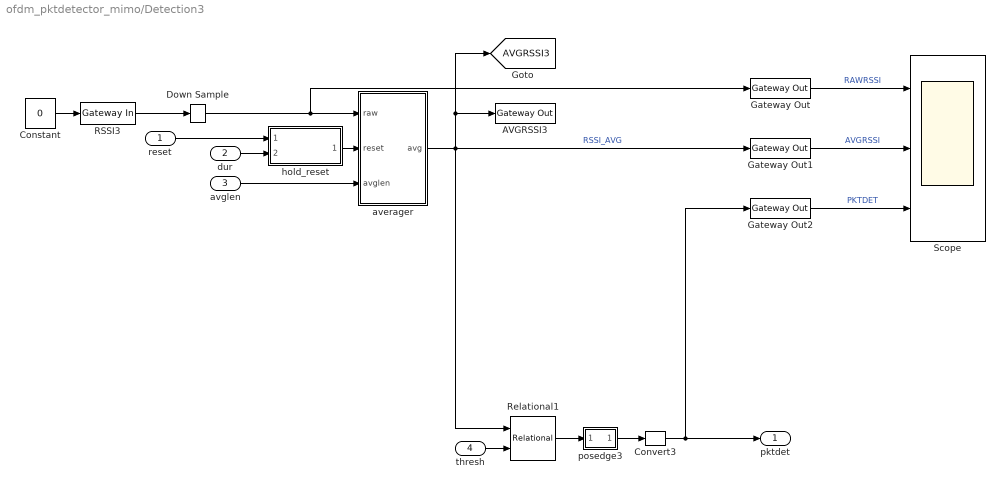
== system ofdm_pktdetector_mimo/Detection3 ==
  reset : Inport
  dur : Inport  Port=2
  avglen : Inport  Port=3
  thresh : Inport  Port=4
  AVGRSSI3 : xbsIndex_r4/Gateway Out  hdl_port=on  timing_constraint=None  locs_specified=off  LOCs={}  block_type=gatewayout
      settings: infoedit="Gateway out block.  Converts Xilinx fixed point inputs into ouputs of type Simulink integer, double, or fixed point.<P><P>Hardware notes:  In hardware these blocks become top level output ports or are discarded, depending on how they are configured."  block_version=8.2
  Constant : Constant  Value=0
  Convert3 : xbsIndex_r4/Convert  arith_type=Unsigned  n_bits=1  bin_pt=0  quantization=Truncate  overflow=Wrap  latency=0  dbl_ovrd=off  pipeline=off  block_type=convert
      settings: block_version=VER_STRING_GOES_HERE
  Down Sample : xbsIndex_r4/Down Sample  sample_ratio=4  sample_phase="Last Value of Frame  (most efficient)"  en=off  latency=1  dbl_ovrd=off  block_type=dsamp
      settings: block_version=VER_STRING_GOES_HERE
  Gateway Out : xbsIndex_r4/Gateway Out  hdl_port=off  timing_constraint=None  locs_specified=off  LOCs={}  block_type=gatewayout
      settings: infoedit="Gateway out block.  Converts Xilinx fixed point inputs into ouputs of type Simulink integer, double, or fixed point.<P><P>Hardware notes:  In hardware these blocks become top level output ports or are discarded, depending on how they are configured."  block_version=8.2
  Gateway Out1 : xbsIndex_r4/Gateway Out  hdl_port=off  timing_constraint=None  locs_specified=off  LOCs={}  block_type=gatewayout
      settings: infoedit="Gateway out block.  Converts Xilinx fixed point inputs into ouputs of type Simulink integer, double, or fixed point.<P><P>Hardware notes:  In hardware these blocks become top level output ports or are discarded, depending on how they are configured."  block_version=8.2
  Gateway Out2 : xbsIndex_r4/Gateway Out  hdl_port=off  timing_constraint=None  locs_specified=off  LOCs={}  block_type=gatewayout
      settings: infoedit="Gateway out block.  Converts Xilinx fixed point inputs into ouputs of type Simulink integer, double, or fixed point.<P><P>Hardware notes:  In hardware these blocks become top level output ports or are discarded, depending on how they are configured."  block_version=8.2
  RSSI3 : xbsIndex_r4/Gateway In  arith_type=Unsigned  n_bits=10  bin_pt=0  quantization="Round  (unbiased: +/- Inf)"  overflow=Saturate  period=1/4  dbl_ovrd=off  timing_constraint=None  locs_specified=off  LOCs={}  block_type=gatewayin
      settings: infoedit="Gateway in block.  Converts inputs of type Simulink integer, double and fixed point to  Xilinx fixed point type.<P><P>Hardware notes:  In hardware these blocks become top level input ports."  block_version=VER_STRING_GOES_HERE
  Relational1 : xbsIndex_r4/Relational  mode=a>b  en=off  latency=0  dbl_ovrd=off  block_type=relational
      settings: block_version=VER_STRING_GOES_HERE
  Scope : Scope  NumInputPorts=3
      settings: YMin=-1~-1~-1  YMax=1~1~1
  averager : Subsystem
  hold_reset : Subsystem
  posedge3 : Subsystem
  pktdet : Outport
  tag scope: AVGRSSI3=global
  wires:
  averager/1(avg) -> Relational1/1, Gateway Out1/1, AVGRSSI3/1, [AVGRSSI3]  "RSSI_AVG"
  hold_reset/1(reset_out) -> averager/2(reset)
  Relational1/1 -> posedge3/1(In)
  posedge3/1(Out) -> Convert3/1
  dur/1 -> hold_reset/2(duration)
  reset/1 -> hold_reset/1(reset_in)
  avglen/1 -> averager/3(avglen)
  Convert3/1 -> pktdet/1, Gateway Out2/1
  thresh/1 -> Relational1/2
  RSSI3/1 -> Down Sample/1
  Down Sample/1 -> averager/1(raw), Gateway Out/1
  Gateway Out/1 -> Scope/1  "RAWRSSI"
  Gateway Out1/1 -> Scope/2  "AVGRSSI"
  Gateway Out2/1 -> Scope/3  "PKTDET"
  Constant/1 -> RSSI3/1

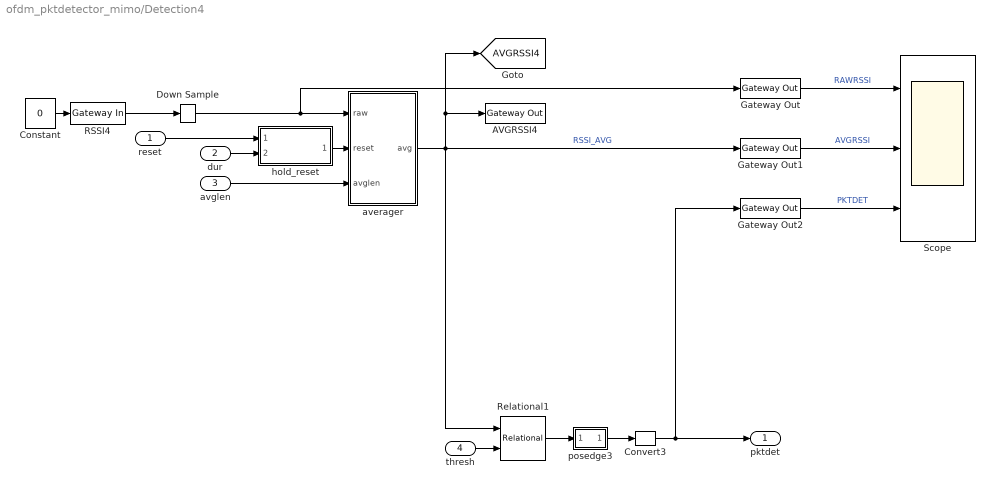
== system ofdm_pktdetector_mimo/Detection4 ==
  reset : Inport
  dur : Inport  Port=2
  avglen : Inport  Port=3
  thresh : Inport  Port=4
  AVGRSSI4 : xbsIndex_r4/Gateway Out  hdl_port=on  timing_constraint=None  locs_specified=off  LOCs={}  block_type=gatewayout
      settings: infoedit="Gateway out block.  Converts Xilinx fixed point inputs into ouputs of type Simulink integer, double, or fixed point.<P><P>Hardware notes:  In hardware these blocks become top level output ports or are discarded, depending on how they are configured."  block_version=8.2
  Constant : Constant  Value=0
  Convert3 : xbsIndex_r4/Convert  arith_type=Unsigned  n_bits=1  bin_pt=0  quantization=Truncate  overflow=Wrap  latency=0  dbl_ovrd=off  pipeline=off  block_type=convert
      settings: block_version=VER_STRING_GOES_HERE
  Down Sample : xbsIndex_r4/Down Sample  sample_ratio=4  sample_phase="Last Value of Frame  (most efficient)"  en=off  latency=1  dbl_ovrd=off  block_type=dsamp
      settings: block_version=VER_STRING_GOES_HERE
  Gateway Out : xbsIndex_r4/Gateway Out  hdl_port=off  timing_constraint=None  locs_specified=off  LOCs={}  block_type=gatewayout
      settings: infoedit="Gateway out block.  Converts Xilinx fixed point inputs into ouputs of type Simulink integer, double, or fixed point.<P><P>Hardware notes:  In hardware these blocks become top level output ports or are discarded, depending on how they are configured."  block_version=8.2
  Gateway Out1 : xbsIndex_r4/Gateway Out  hdl_port=off  timing_constraint=None  locs_specified=off  LOCs={}  block_type=gatewayout
      settings: infoedit="Gateway out block.  Converts Xilinx fixed point inputs into ouputs of type Simulink integer, double, or fixed point.<P><P>Hardware notes:  In hardware these blocks become top level output ports or are discarded, depending on how they are configured."  block_version=8.2
  Gateway Out2 : xbsIndex_r4/Gateway Out  hdl_port=off  timing_constraint=None  locs_specified=off  LOCs={}  block_type=gatewayout
      settings: infoedit="Gateway out block.  Converts Xilinx fixed point inputs into ouputs of type Simulink integer, double, or fixed point.<P><P>Hardware notes:  In hardware these blocks become top level output ports or are discarded, depending on how they are configured."  block_version=8.2
  RSSI4 : xbsIndex_r4/Gateway In  arith_type=Unsigned  n_bits=10  bin_pt=0  quantization="Round  (unbiased: +/- Inf)"  overflow=Saturate  period=1/4  dbl_ovrd=off  timing_constraint=None  locs_specified=off  LOCs={}  block_type=gatewayin
      settings: infoedit="Gateway in block.  Converts inputs of type Simulink integer, double and fixed point to  Xilinx fixed point type.<P><P>Hardware notes:  In hardware these blocks become top level input ports."  block_version=VER_STRING_GOES_HERE
  Relational1 : xbsIndex_r4/Relational  mode=a>b  en=off  latency=0  dbl_ovrd=off  block_type=relational
      settings: block_version=VER_STRING_GOES_HERE
  Scope : Scope  NumInputPorts=3
      settings: YMin=-1~-1~-1  YMax=1~1~1
  averager : Subsystem
  hold_reset : Subsystem
  posedge3 : Subsystem
  pktdet : Outport
  tag scope: AVGRSSI4=global
  wires:
  Gateway Out2/1 -> Scope/3  "PKTDET"
  Gateway Out1/1 -> Scope/2  "AVGRSSI"
  Gateway Out/1 -> Scope/1  "RAWRSSI"
  Down Sample/1 -> Gateway Out/1, averager/1(raw)
  RSSI4/1 -> Down Sample/1
  thresh/1 -> Relational1/2
  Convert3/1 -> Gateway Out2/1, pktdet/1
  avglen/1 -> averager/3(avglen)
  reset/1 -> hold_reset/1(reset_in)
  dur/1 -> hold_reset/2(duration)
  posedge3/1(Out) -> Convert3/1
  Relational1/1 -> posedge3/1(In)
  hold_reset/1(reset_out) -> averager/2(reset)
  averager/1(avg) -> [AVGRSSI4], AVGRSSI4/1, Gateway Out1/1, Relational1/1  "RSSI_AVG"
  Constant/1 -> RSSI4/1
